simulink model "HDLOFDMSS"  (R2024a)
settings: Solver=FixedStepDiscrete  StartTime=0.0  StopTime=stopTime  RelTol=1e-3
undefined symbols (not defined in the file or in its folder): CONST
libraries: dspsrcs4 x2, HDL_ieee_8021513 x2, hdlsllib x1, whdlutilities x1
settings Model: DataTypeOverride=Off  SimulationMode=accelerator  Creator=cotti  LastModifiedBy=cotti
settings OptimizationCC: BlockReduction=off  ConditionallyExecuteInputs=off  DefaultParameterBehavior=Inlined  InheritOutputTypeSmallerThanSingle=on
settings DebuggingCC: AlgebraicLoopMsg=error  ArtificialAlgebraicLoopMsg=error  SingleTaskRateTransMsg=error  UnconnectedInputMsg=warning  UnconnectedOutputMsg=warning  UnconnectedLineMsg=warning
settings HardwareCC: ProdBitPerPointer=32  ProdBitPerSizeT=32  ProdBitPerPtrDiffT=32  ProdLargestAtomicFloat=None  ProdIntDivRoundTo=Undefined  ProdEndianess=Unspecified  ProdWordSize=32  ProdHWDeviceType=ASIC/FPGA->ASIC/FPGA  TargetBitPerLong=64  TargetBitPerPointer=64  TargetBitPerSizeT=64  TargetBitPerPtrDiffT=64  TargetLongLongMode=on  TargetIntDivRoundTo=Zero  TargetEndianess=LittleEndian  TargetWordSize=64  TargetHWDeviceType=Custom Processor->MATLAB Host Computer  ProdEqTarget=off

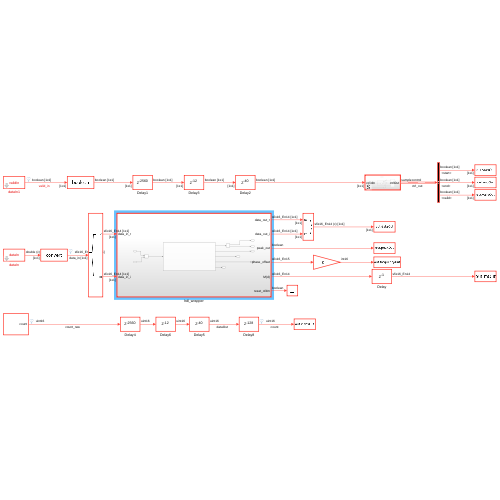
[thumbnail: Simulink's stored preview of the top-level diagram]
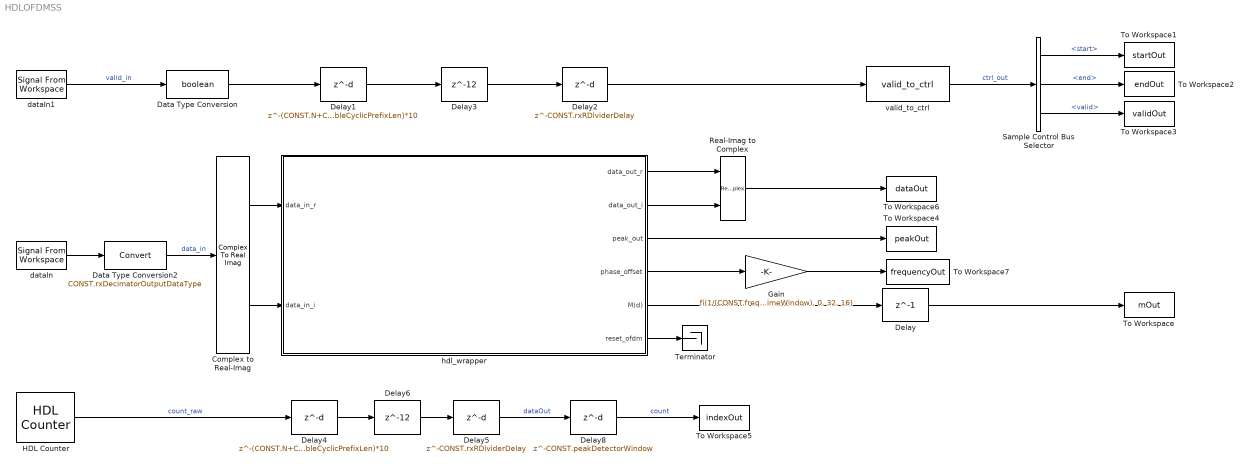
== system HDLOFDMSS ==
  Complex to Real-Imag : ComplexToRealImag
  Data Type Conversion : DataTypeConversion  OutDataTypeStr=boolean  SaturateOnIntegerOverflow=off  RndMeth=Floor
  Data Type Conversion2 : DataTypeConversion  OutDataTypeStr=CONST.rxDecimatorOutputDataType  SaturateOnIntegerOverflow=off  RndMeth=Floor
  Delay : Delay  DelayLength=1  InitialCondition=0  UseCircularBuffer=on
  Delay1 : Delay  DelayLength=(CONST.N+CONST.preambleCyclicPrefixLen)*10  InitialCondition=0  UseCircularBuffer=on
  Delay2 : Delay  DelayLength=CONST.rxRDividerDelay  InitialCondition=0  UseCircularBuffer=on
  Delay3 : Delay  DelayLength=12  InitialCondition=0  UseCircularBuffer=on
  Delay4 : Delay  DelayLength=(CONST.N+CONST.preambleCyclicPrefixLen)*10  InitialCondition=0  UseCircularBuffer=on
  Delay5 : Delay  DelayLength=CONST.rxRDividerDelay  InitialCondition=0  UseCircularBuffer=on
  Delay6 : Delay  DelayLength=12  InitialCondition=0  UseCircularBuffer=on
  Delay8 : Delay  DelayLength=CONST.peakDetectorWindow  InitialCondition=0  UseCircularBuffer=on
  Gain : Gain  Gain=fi(1/(CONST.frequencyOffsetTimeWindow), 0, 32, 16)  ParamDataTypeStr=fixdt(0,32,16)  OutDataTypeStr=int16
  HDL Counter : hdlsllib/Sources/HDL Counter  CountType=Free running  CountInit=0  CountStep=1  CountMax=25  CountFromType=Initial value  CountFrom=0  CountResetPort=off  CountLoadPort=off  CountEnbPort=off  CountDirPort=off  CountHitOutputPort=off  CountDataType=Unsigned  CountWordLen=16  CountFracLen=0  CountSampTime=1/CONST.fPHY
  Real-Imag to Complex : RealImagToComplex
  Sample Control Bus Selector : whdlutilities/Sample Control Bus Selector  OutputSignals=start,end,valid
  Terminator : Terminator
  To Workspace : ToWorkspace  VariableName=mOut  SampleTime=1/CONST.fPHY
      settings: Save2DSignal=2-D array (concatenate along first dimension)
  To Workspace1 : ToWorkspace  VariableName=startOut  SampleTime=1/CONST.fPHY
      settings: Save2DSignal=2-D array (concatenate along first dimension)
  To Workspace2 : ToWorkspace  VariableName=endOut  SampleTime=1/CONST.fPHY
      settings: Save2DSignal=2-D array (concatenate along first dimension)
  To Workspace3 : ToWorkspace  VariableName=validOut  SampleTime=1/CONST.fPHY
      settings: Save2DSignal=2-D array (concatenate along first dimension)
  To Workspace4 : ToWorkspace  VariableName=peakOut  SampleTime=1/CONST.fPHY
      settings: Save2DSignal=2-D array (concatenate along first dimension)
  To Workspace5 : ToWorkspace  VariableName=indexOut  SampleTime=1/CONST.fPHY
      settings: Save2DSignal=2-D array (concatenate along first dimension)
  To Workspace6 : ToWorkspace  VariableName=dataOut  SampleTime=1/CONST.fPHY
      settings: Save2DSignal=2-D array (concatenate along first dimension)
  To Workspace7 : ToWorkspace  VariableName=frequencyOut  SampleTime=1/CONST.fPHY
      settings: Save2DSignal=2-D array (concatenate along first dimension)
  dataIn : dspsrcs4/Signal From Workspace  X=dataIn  Ts=1/CONST.fPHY  nsamps=1  OutputAfterFinalValue=Setting to zero  ignoreOrWarnInputAndFrameLengths=off  OutputFrames=off
  dataIn1 : dspsrcs4/Signal From Workspace  X=validIn  Ts=1/CONST.fPHY  nsamps=1  OutputAfterFinalValue=Setting to zero  ignoreOrWarnInputAndFrameLengths=off  OutputFrames=off
  hdl_wrapper : Subsystem  TreatAsAtomicUnit=on
  valid_to_ctrl : HDL_ieee_8021513/valid_to_ctrl  SystemSampleTime=-1  VariantActivationTime=update diagram  AllowFlexibleInterface=on  Latency=0  AutoFrameSizeCalculation=off
      settings: SourceProductName=HDL IEEE 8021513
  wires:
  Sample Control Bus Selector/2 -> To Workspace2/1  "<end>"
  Sample Control Bus Selector/3 -> To Workspace3/1  "<valid>"
  Sample Control Bus Selector/1 -> To Workspace1/1  "<start>"
  valid_to_ctrl/1 -> Sample Control Bus Selector/1  "ctrl_out"
  dataIn1/1 -> Data Type Conversion/1  "valid_in"
  Delay2/1 -> valid_to_ctrl/1
  Data Type Conversion/1 -> Delay1/1
  Delay1/1 -> Delay3/1
  Delay3/1 -> Delay2/1
  Delay4/1 -> Delay6/1
  Delay6/1 -> Delay5/1
  HDL Counter/1 -> Delay4/1  "count_raw"
  Delay5/1 -> Delay8/1  "dataOut"
  Delay/1 -> To Workspace/1
  dataIn/1 -> Data Type Conversion2/1
  Delay8/1 -> To Workspace5/1  "count"
  Gain/1 -> To Workspace7/1
  hdl_wrapper/3(peak_out) -> To Workspace4/1
  hdl_wrapper/4(phase_offset) -> Gain/1
  hdl_wrapper/5(M(d)) -> Delay/1
  hdl_wrapper/6(reset_ofdm) -> Terminator/1
  hdl_wrapper/1(data_out_r) -> Real-Imag to Complex/1
  hdl_wrapper/2(data_out_i) -> Real-Imag to Complex/2
  Real-Imag to Complex/1 -> To Workspace6/1
  Data Type Conversion2/1 -> Complex to Real-Imag/1  "data_in"
  Complex to Real-Imag/1 -> hdl_wrapper/1(data_in_r)
  Complex to Real-Imag/2 -> hdl_wrapper/2(data_in_i)

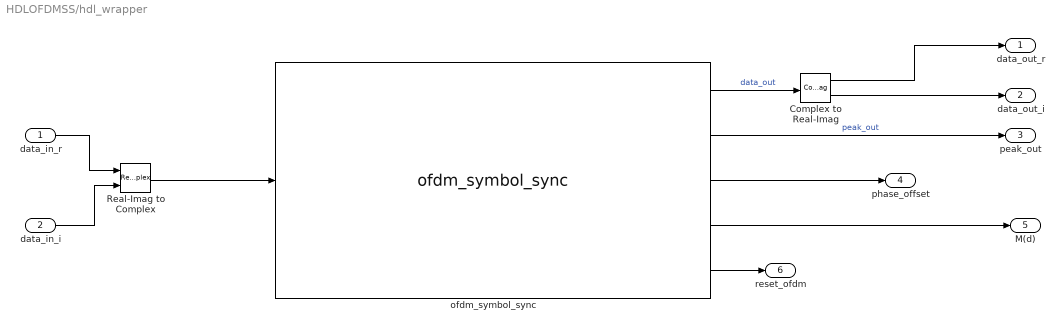
== system HDLOFDMSS/hdl_wrapper ==
  data_in_r : Inport
  data_in_i : Inport  Port=2
  Complex to Real-Imag : ComplexToRealImag
  Real-Imag to Complex : RealImagToComplex
  ofdm_symbol_sync : HDL_ieee_8021513/ofdm_symbol_sync  SystemSampleTime=-1  VariantActivationTime=update diagram  AllowFlexibleInterface=on  Latency=0  AutoFrameSizeCalculation=off
      settings: SourceProductName=HDL IEEE 8021513
  data_out_r : Outport
  data_out_i : Outport  Port=2
  peak_out : Outport  Port=3
  phase_offset : Outport  Port=4
  M(d) : Outport  Port=5
  reset_ofdm : Outport  Port=6
  wires:
  ofdm_symbol_sync/2 -> peak_out/1  "peak_out"
  ofdm_symbol_sync/3 -> phase_offset/1
  ofdm_symbol_sync/4 -> M(d)/1
  ofdm_symbol_sync/5 -> reset_ofdm/1
  data_in_r/1 -> Real-Imag to Complex/1
  data_in_i/1 -> Real-Imag to Complex/2
  Real-Imag to Complex/1 -> ofdm_symbol_sync/1
  ofdm_symbol_sync/1 -> Complex to Real-Imag/1  "data_out"
  Complex to Real-Imag/1 -> data_out_r/1
  Complex to Real-Imag/2 -> data_out_i/1
